simulink model "StateSpace"  (R2020b)
settings: Solver=VariableStepAuto  StartTime=0.0  StopTime=10.0  RelTol=1e-3
values from neighbouring files (symbols this model uses):
  K = place(A,B,P)    [calculate.m]
  kp = wn^2    (= 100)    [calculate.m]
undefined symbols (not defined in the file or in its folder): A, B, C
settings Model: Creator=huang  LastModifiedBy=huang

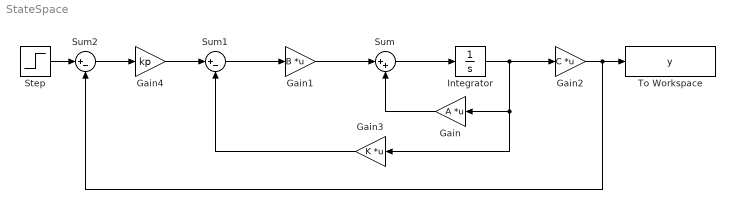
== system StateSpace ==
  Gain : Gain  Gain=A  Multiplication=Matrix(K*u)
  Gain1 : Gain  Gain=B  Multiplication=Matrix(K*u)
  Gain2 : Gain  Gain=C  Multiplication=Matrix(K*u)
  Gain3 : Gain  Gain=K  Multiplication=Matrix(K*u)
  Gain4 : Gain  Gain=kp
  Integrator : Integrator
  Step : Step  Time=0  SampleTime=0
  Sum : Sum  Inputs=|++
  Sum1 : Sum  Inputs=|+-
  Sum2 : Sum  Inputs=|+-
  To Workspace : ToWorkspace  VariableName=y  SampleTime=-1
      settings: Save2DSignal=2-D array (concatenate along first dimension)
  wires:
  Gain1/1 -> Sum/1
  Gain/1 -> Sum/2
  Sum/1 -> Integrator/1
  Integrator/1 -> Gain2/1, Gain3/1, Gain/1
  Gain2/1 -> Sum2/2, To Workspace/1
  Sum1/1 -> Gain1/1
  Gain3/1 -> Sum1/2
  Step/1 -> Sum2/1
  Gain4/1 -> Sum1/1
  Sum2/1 -> Gain4/1
